simulink model "test_serial"  (R2016a)
settings: Solver=FixedStepDiscrete  StartTime=0.0  StopTime=50.0  RelTol=1e-3
libraries: c280xlib x2, c2837xDlib x1
settings Model: SimulationMode=external  ExtModeTrigDuration=8  Creator=ric  LastModifiedBy=ric
settings OptimizationCC: OptimizeModelRefInitCode=on  LifeSpan=1  MaxStackSize=512
settings HardwareCC: ProdBitPerChar=16  ProdBitPerInt=16  ProdBitPerPointer=32  ProdLargestAtomicInteger=Integer  ProdLargestAtomicFloat=None  ProdWordSize=16  ProdLongLongMode=on  ProdHWDeviceType=Texas Instruments->C2000
settings RTWCC: SystemTargetFile=ert.tlc  HardwareBoard=TI Delfino F2837xS  TemplateMakefile=ert_default_tmf  GenerateReport=on  RTWVerbose=off  Toolchain=Texas Instruments Code Composer Studio v6 (C2000)  IncludeHyperlinkInReport=on  LaunchReport=on  GenerateTraceInfo=on  GenerateTraceReport=on  GenerateTraceReportSl=on  GenerateTraceReportSf=on  GenerateTraceReportEml=on
settings CodeAppCC: ForceParamTrailComments=on  IgnoreCustomStorageClasses=off  OperatorAnnotations=on  SimulinkDataObjDesc=on  SFDataObjDesc=on  MATLABFcnDesc=on  InsertBlockDesc=on  MATLABSourceComments=on
settings ERTTargetCC: CodeReplacementLibrary=TI C28x

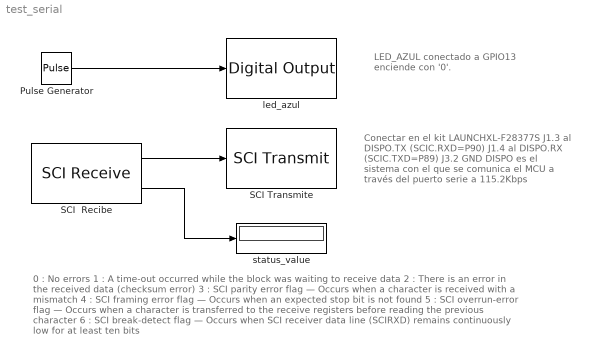
== system test_serial ==
  note: 0 : No errors
      | 1 : A time-out occurred while the block was waiting to receive data
      | 2 : There is an error in the received data (checksum error)
      | 3 : SCI parity error flag — Occurs when a character is received with a mismatch
      | 4 : SCI framing error flag — Occurs when an expected stop bit is not found
      | 5 : SCI overrun-error flag — Occurs when a character is transferred to the receive registers before reading the previous character
      | 6 : SCI break-detect flag — Occurs when SCI receiver data line (SCIRXD) remains continuously low for at least ten bits
  note: LED_AZUL conectado a GPIO13
      | enciende con '0'.
  note: Conectar en el kit LAUNCHXL-F28377S
      | J1.3 al DISPO.TX (SCIC.RXD=P90)
      | J1.4 al DISPO.RX (SCIC.TXD=P89)
      | J3.2 GND
      | DISPO es el sistema con el que se
      | comunica el MCU a través del puerto
      | serie a 115.2Kbps
  Pulse Generator : DiscretePulseGenerator  PulseType=Time based  Period=1  PulseWidth=50
  SCI  Recibe : c280xlib/SCI Receive  sciModule=C  dataHead=''  dataTail=''  dataType=uint8  dataDim=1  initValue=0  errOption=Output custom value  errValue=0  sampleTime=0.01  outputStatus=on  postInterrupt=off  numFifo=1
  SCI Transmite : c280xlib/SCI Transmit  sciModule=C  dataHead=''  dataTail=''  postInterrupt=off  numFifo=1
  led_azul : c2837xDlib/Digital Output  GPIO_Number=GPIO8~GPIO15  GPIO_Bit0=off  GPIO_BIT0_Toggle=off  GPIO_Bit1=off  GPIO_BIT1_Toggle=off  GPIO_Bit2=off  GPIO_BIT2_Toggle=off  GPIO_Bit3=off  GPIO_BIT3_Toggle=off  GPIO_Bit4=off  GPIO_BIT4_Toggle=off  GPIO_Bit5=on  GPIO_BIT5_Toggle=off  GPIO_Bit6=off  GPIO_BIT6_Toggle=off  GPIO_Bit7=off  GPIO_BIT7_Toggle=off
  status_value : Display
  wires:
  Pulse Generator/1 -> led_azul/1
  SCI  Recibe/1 -> SCI Transmite/1
  SCI  Recibe/2 -> status_value/1
